simulink model "simplified_STG"  (R2022a)
settings: Solver=VariableStepAuto  StartTime=0.0  StopTime=30  FixedStep=1e-4  RelTol=1e-3
model workspace (MAT data in the model file):
  a = 0.01
  gsyn_base = -1
  loss_prob = 0
libraries: neuromorphic_blocks x11
settings Model: SimulationMode=rapid-accelerator  Creator=chris  LastModifiedBy=chris
settings OptimizationCC: ZeroExternalMemoryAtStartup=off  ZeroInternalMemoryAtStartup=off  InitFltsAndDblsToZero=on  SimCompilerOptimization=on
settings HardwareCC: ProdLongLongMode=on  TargetLongLongMode=on
settings SFSimCC: SimHardwareAcceleration=native  SimTargetLang=C++
settings RTWCC: BuildConfiguration=Faster Runs  TargetLang=C++  GenerateGPUCode=CUDA
settings GRTTargetCC: TargetLangStandard=C++11 (ISO)  CodeInterfacePackaging=C++ class

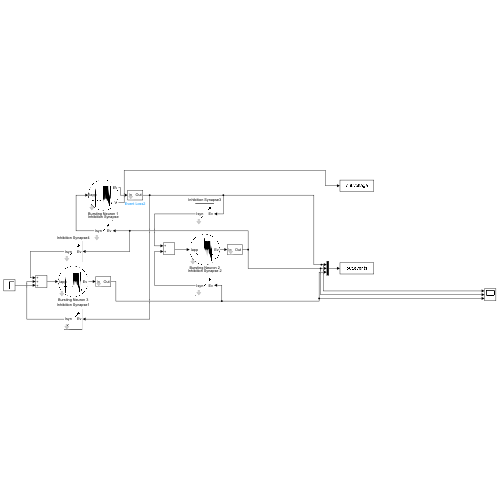
[thumbnail: Simulink's stored preview of the top-level diagram]
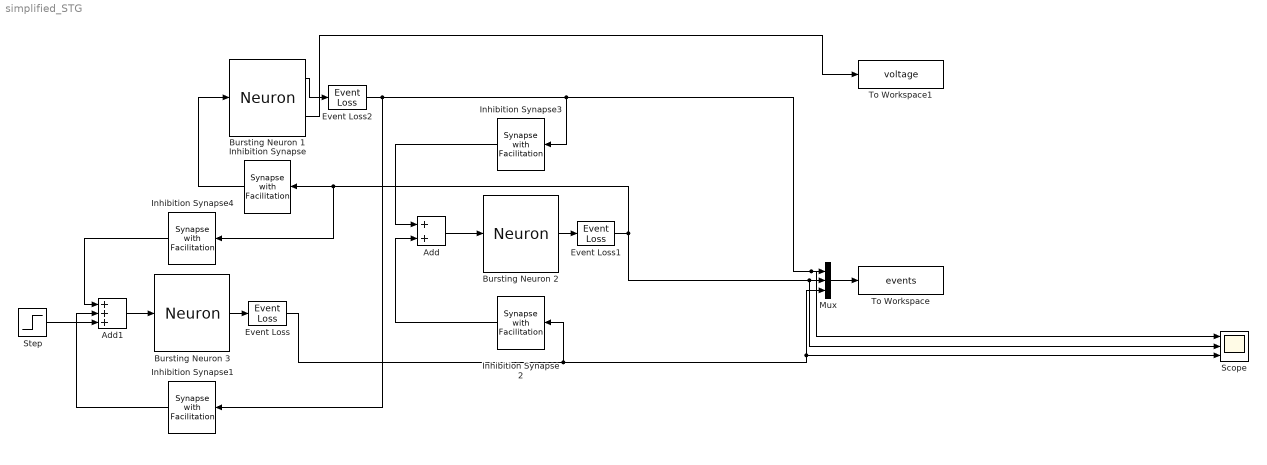
== system simplified_STG ==
  Add : Sum
  Add1 : Sum  Inputs=+++
  Bursting Neuron 1 : neuromorphic_blocks/Neural Blocks/Neuron  gfm_source=Internal  gfm=3  gsp_source=Internal  gsp=6  gsm_source=Internal  gsm=2.5  gup_source=Internal  gup=5  gum_source=Internal  gum=2  dfm=0  dsp=0.5  dsm=-0.5  dup=-0.5  dum=-1  mfm=1  msp=1  msm=1  mup=1  mum=1  timescale=0.004  rel_membrane=0.1  rel_fast=0.1  rel_slow=4  rel_ultraslow=200  Iapp_base=0.1  V0=-1.2  tresh=0  output=Both
      settings: SourceProductName=Neuromorphic Toolbox
  Bursting Neuron 2 : neuromorphic_blocks/Neural Blocks/Neuron  gfm_source=Internal  gfm=3  gsp_source=Internal  gsp=6  gsm_source=Internal  gsm=2.5  gup_source=Internal  gup=5  gum_source=Internal  gum=2  dfm=0  dsp=0.5  dsm=-0.5  dup=-0.5  dum=-1  mfm=1  msp=1  msm=1  mup=1  mum=1  timescale=0.004  rel_membrane=0.1  rel_fast=0.1  rel_slow=4  rel_ultraslow=200  Iapp_base=0.1  V0=-1.2  tresh=0  output=Events
      settings: SourceProductName=Neuromorphic Toolbox
  Bursting Neuron 3 : neuromorphic_blocks/Neural Blocks/Neuron  gfm_source=Internal  gfm=3  gsp_source=Internal  gsp=6  gsm_source=Internal  gsm=2.5  gup_source=Internal  gup=5  gum_source=Internal  gum=2  dfm=0  dsp=0.5  dsm=-0.5  dup=-0.5  dum=-1  mfm=1  msp=1  msm=1  mup=1  mum=1  timescale=0.004  rel_membrane=0.1  rel_fast=0.1  rel_slow=4  rel_ultraslow=200  Iapp_base=0.1  V0=-1.2  tresh=0  output=Events
      settings: SourceProductName=Neuromorphic Toolbox
  Event Loss : neuromorphic_blocks/Events Transmission Blocks/Event Loss  loss_prob=loss_prob  seed=-1  seed_mem=randi([0, 100000])
      settings: SourceProductName=Neuromorphic Toolbox
  Event Loss1 : neuromorphic_blocks/Events Transmission Blocks/Event Loss  loss_prob=loss_prob  seed=-1  seed_mem=randi([0, 100000])
      settings: SourceProductName=Neuromorphic Toolbox
  Event Loss2 : neuromorphic_blocks/Events Transmission Blocks/Event Loss  loss_prob=loss_prob  seed=-1  seed_mem=randi([0, 100000])
      settings: SourceProductName=Neuromorphic Toolbox
  Inhibition Synapse : neuromorphic_blocks/Neural Blocks/Synapse with Facilitation  gsyn_source=Internal  gsyn=gsyn_base  dsyn=4  msyn=10  timescale=0.004  rel_timescale=10  input=Events  gsyn_in=0  dsyn_in=0  msyn_in=1
      settings: SourceProductName=Neuromorphic Toolbox
  Inhibition Synapse 2 : neuromorphic_blocks/Neural Blocks/Synapse with Facilitation  gsyn_source=Internal  gsyn=gsyn_base  dsyn=4  msyn=10  timescale=0.004  rel_timescale=10  input=Events  gsyn_in=0  dsyn_in=0  msyn_in=1
      settings: SourceProductName=Neuromorphic Toolbox
  Inhibition Synapse1 : neuromorphic_blocks/Neural Blocks/Synapse with Facilitation  gsyn_source=Internal  gsyn=gsyn_base  dsyn=4  msyn=10  timescale=0.004  rel_timescale=10  input=Events  gsyn_in=0  dsyn_in=0  msyn_in=1
      settings: SourceProductName=Neuromorphic Toolbox
  Inhibition Synapse3 : neuromorphic_blocks/Neural Blocks/Synapse with Facilitation  gsyn_source=Internal  gsyn=gsyn_base*a  dsyn=4  msyn=10  timescale=0.004  rel_timescale=10  input=Events  gsyn_in=0  dsyn_in=0  msyn_in=1
      settings: SourceProductName=Neuromorphic Toolbox
  Inhibition Synapse4 : neuromorphic_blocks/Neural Blocks/Synapse with Facilitation  gsyn_source=Internal  gsyn=gsyn_base*a  dsyn=4  msyn=10  timescale=0.004  rel_timescale=10  input=Events  gsyn_in=0  dsyn_in=0  msyn_in=1
      settings: SourceProductName=Neuromorphic Toolbox
  Mux : Mux  Inputs=3
  Scope : Scope  NumInputPorts=3
  Step : Step  Before=-1  After=0  SampleTime=0
  To Workspace : ToWorkspace  VariableName=events  SaveFormat=Structure With Time  SampleTime=-1
  To Workspace1 : ToWorkspace  VariableName=voltage  SaveFormat=Structure With Time  SampleTime=-1
  wires:
  Bursting Neuron 3/1 -> Event Loss/1
  Inhibition Synapse/1 -> Bursting Neuron 1/1
  Bursting Neuron 2/1 -> Event Loss1/1
  Bursting Neuron 1/1 -> Event Loss2/1
  Add/1 -> Bursting Neuron 2/1
  Inhibition Synapse 2/1 -> Add/2
  Inhibition Synapse3/1 -> Add/1
  Add1/1 -> Bursting Neuron 3/1
  Inhibition Synapse1/1 -> Add1/2
  Inhibition Synapse4/1 -> Add1/1
  Step/1 -> Add1/3
  Mux/1 -> To Workspace/1
  Bursting Neuron 1/2 -> To Workspace1/1
  Event Loss2/1 -> Inhibition Synapse1/1, Inhibition Synapse3/1, Scope/1, Mux/1
  Event Loss1/1 -> Scope/2, Mux/2, Inhibition Synapse4/1, Inhibition Synapse/1
  Event Loss/1 -> Scope/3, Mux/3, Inhibition Synapse 2/1
